simulink model "cpg_2015"  (R2015b)
settings: Solver=ode1  StartTime=0.0  StopTime=3  FixedStep=0.001  RelTol=1e-3
undefined symbols (not defined in the file or in its folder): DiscIntNeverNeededParam
settings Model: Creator=KAREN  LastModifiedBy=rodri

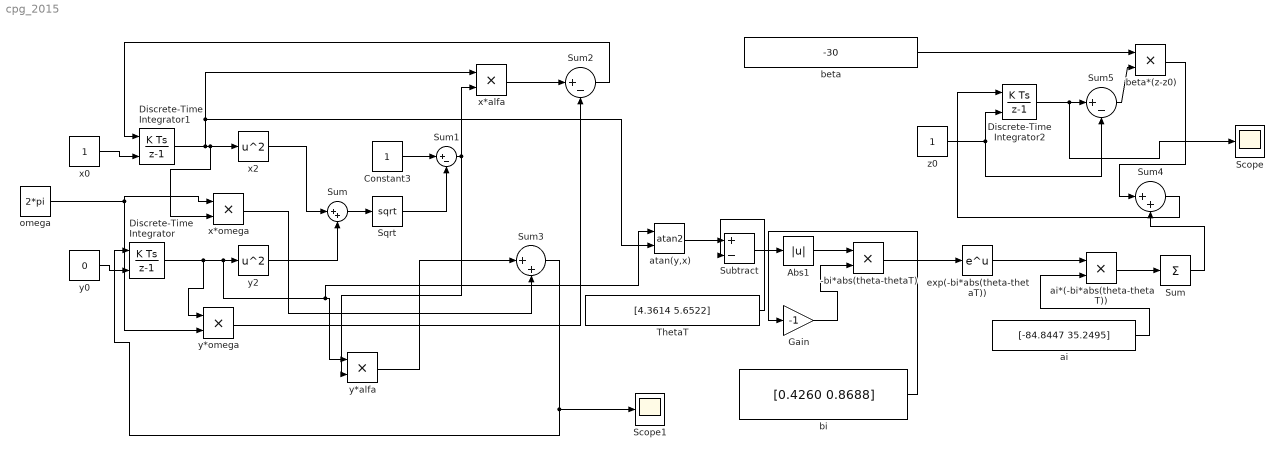
== system cpg_2015 ==
  -bi*abs(theta-thetaT) : Product
  Abs1 : Abs
  Constant3 : Constant
  Discrete-Time Integrator : DiscreteIntegrator  InitialConditionSource=external  InitialConditionSetting=State (most efficient)  SampleTime=0.001  ICPrevOutput=DiscIntNeverNeededParam  ICPrevScaledInput=DiscIntNeverNeededParam
  Discrete-Time Integrator1 : DiscreteIntegrator  InitialConditionSource=external  InitialConditionSetting=State (most efficient)  SampleTime=0.001  ICPrevOutput=DiscIntNeverNeededParam  ICPrevScaledInput=DiscIntNeverNeededParam
  Discrete-Time Integrator2 : DiscreteIntegrator  InitialConditionSource=external  InitialConditionSetting=State (most efficient)  SampleTime=0.001  ICPrevOutput=DiscIntNeverNeededParam  ICPrevScaledInput=DiscIntNeverNeededParam
  Gain : Gain  Gain=-1
  Scope : Scope
  Scope1 : Scope
  Sqrt : Sqrt  SaturateOnIntegerOverflow=on
  Subtract : Sum  Inputs=+-
  Sum : Sum  Inputs=|++
  "Sum " : Sum  Inputs=+
  Sum1 : Sum  Inputs=|+-
  Sum2 : Sum  Inputs=|+-
  Sum3 : Sum  Inputs=|++
  Sum4 : Sum  Inputs=|++
  Sum5 : Sum  Inputs=|+-
  ThetaT : Constant  Value=[4.3614 5.6522]
  ai : Constant  Value=[-84.8447 35.2495]
  ai*(-bi*abs(theta-thetaT)) : Product
  atan(y,x) : Trigonometry  Operator=atan2
  beta : Constant  Value=-30
  beta*(z-z0) : Product
  bi : Constant  Value=[0.4260 0.8688]
  exp(-bi*abs(theta-thetaT)) : Math  SaturateOnIntegerOverflow=on
  omega : Constant  Value=2*pi
  x*alfa : Product
  x*omega : Product
  x0 : Constant
  x2 : Math  Operator=square  SaturateOnIntegerOverflow=on
  y*alfa : Product
  y*omega : Product
  y0 : Constant  Value=0
  y2 : Math  Operator=square  SaturateOnIntegerOverflow=on
  z0 : Constant
  wires:
  x0/1 -> Discrete-Time Integrator1/2
  y0/1 -> Discrete-Time Integrator/2
  Discrete-Time Integrator1/1 -> x*alfa/1, atan(y,x)/2, x*omega/2, x2/1
  x2/1 -> Sum/1
  y2/1 -> Sum/2
  Sum/1 -> Sqrt/1
  Sqrt/1 -> Sum1/2
  Constant3/1 -> Sum1/1
  omega/1 -> y*omega/2, x*omega/1
  Sum1/1 -> x*alfa/2, y*alfa/2
  y*omega/1 -> Sum2/2
  x*alfa/1 -> Sum2/1
  Sum2/1 -> Discrete-Time Integrator1/1
  y*alfa/1 -> Sum3/1
  x*omega/1 -> Sum3/2
  Sum3/1 -> Discrete-Time Integrator/1, Scope1/1
  Discrete-Time Integrator/1 -> y*omega/1, atan(y,x)/1, y*alfa/1, y2/1
  atan(y,x)/1 -> Subtract/1
  ThetaT/1 -> Subtract/2
  Subtract/1 -> Abs1/1
  Abs1/1 -> -bi*abs(theta-thetaT)/1
  bi/1 -> Gain/1
  Gain/1 -> -bi*abs(theta-thetaT)/2
  -bi*abs(theta-thetaT)/1 -> exp(-bi*abs(theta-thetaT))/1
  exp(-bi*abs(theta-thetaT))/1 -> ai*(-bi*abs(theta-thetaT))/1
  ai/1 -> ai*(-bi*abs(theta-thetaT))/2
  ai*(-bi*abs(theta-thetaT))/1 -> "Sum "/1
  "Sum "/1 -> Sum4/2
  z0/1 -> Discrete-Time Integrator2/2, Sum5/2
  Discrete-Time Integrator2/1 -> Scope/1, Sum5/1
  Sum5/1 -> beta*(z-z0)/2
  beta*(z-z0)/1 -> Sum4/1
  Sum4/1 -> Discrete-Time Integrator2/1
  beta/1 -> beta*(z-z0)/1
